simulink model "sf_tictacflow"  (R2017b)
settings: Solver=VariableStepDiscrete  StartTime=0.0  StopTime=inf  RelTol=1e-3  EnableMultiTasking=on
settings Model: FPTRunName=Active  ExtModeTrigMode=oneshot  ExtModeArmWhenConnect=off  ExtModeAutoUpdateStatusClock=off  Creator=The MathWorks, Inc.  LastModifiedBy=The MathWorks, Inc.
settings DataIOCC: SaveFormat=Array  SaveOutput=off  SaveTime=off  SignalLoggingName=sigsOut
settings OptimizationCC: BlockReduction=off  BooleanDataType=off  ExpressionDepthLimit=2147483647  InitFltsAndDblsToZero=on  EfficientMapNaN2IntZero=off  LifeSpan=inf  BufferReusableBoundary=off
settings DebuggingCC: SaveWithParameterizedLinksMsg=none  UnderspecifiedInitializationDetection=Classic  MergeDetectMultiDrivingBlocksExec=none  SignalResolutionControl=TryResolveAllWithWarning  MultiTaskDSMMsg=warning  MultiTaskCondExecSysMsg=none  FcnCallInpInsideContextMsg=warning  BusObjectLabelMismatch=none  AllowSymbolicDim=off  StateNameClashWarn=warning  SFUnexpectedBacktrackingDiag=warning  SFInvalidInputDataAccessInChartInitDiag=none  SFNoUnconditionalDefaultTransitionDiag=warning  SFUndirectedBroadcastEventsDiag=none  SFExecutionAtInitializationDiag=none  SFMachineParentedDataDiag=none
settings HardwareCC: ProdBitPerPointer=32  ProdBitPerSizeT=32  ProdBitPerPtrDiffT=32  ProdLargestAtomicFloat=None  ProdIntDivRoundTo=Undefined  ProdEndianess=Unspecified  ProdWordSize=32  ProdHWDeviceType=32-bit Generic  TargetUnknown=on
settings ModelReferenceCC: PropagateSignalLabelsOutOfModel=off
settings SFSimCC: SFSimEcho=off  SimParseCustomCode=off
settings CodeAppCC: StateflowObjectComments=on
settings GRTTargetCC: TargetFcnLib=ansi_tfl_tmw.mat  TargetLangStandard=C89/C90 (ANSI)  GeneratePreprocessorConditionals=Disable all  CombineOutputUpdateFcns=off  GRTInterface=on
settings ConfigComp: CovMetricSettings=dcmtr  CovHtmlReporting=on  CovSaveCumulativeToWorkspaceVar=on  CovSaveSingleToWorkspaceVar=on  CovExternalEMLEnable=off  CovSFcnEnable=off

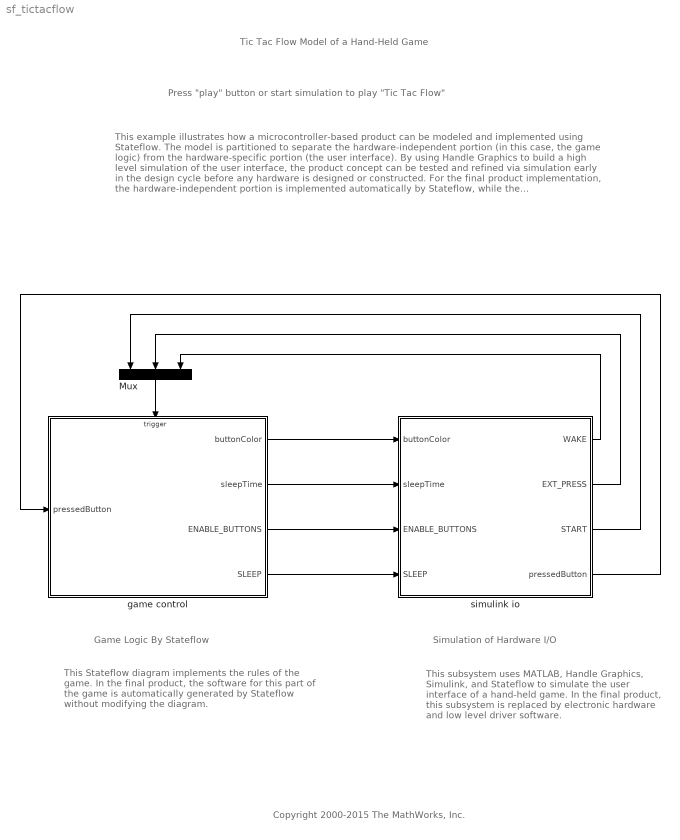
== system sf_tictacflow ==
  note: Press "play" button or start simulation to play "Tic Tac Flow"
  note: This Stateflow diagram implements
      | the rules of the game.
      |
      | In the final product, the software for this
      | part of the game is automatically generated
      |  by Stateflow without modifying the diagram.
  note: Game Logic By Stateflow
  note: This subsystem uses MATLAB, Handle
      | Graphics, Simulink, and Stateflow
      |  to simulate the user interface of a
      | hand-held game.
      |
      | In the final product, this subsystem is
      | replaced by electronic hardware and
      | low level driver software.
  note: This example illustrates how a microcontroller-based product can be modeled and implemented using Stateflow.
      |
      | The model is partitioned to separate the hardware-independent portion (in
      | this case, the game logic) from the hardware-specific portion (the user interface).
      | By using Handle Graphics to build a high level simulation of the user interface, the product concept can
      |  be tested and refined via simulation early in the design cycle before any hardware is designed or constructed.
      | For the final product implementation, the hardware-independent portion is implemented automatically
      |  by Stateflow, while the hardware-specific portion is replaced by actual hardware and low-level driver software.
  note: Tic Tac Flow
      | Model of a Hand-Held Game
  note: Simulation of Hardware I/O
  note: Copyright 2000-2015 The MathWorks, Inc.
  Mux : Mux  Inputs=3
  game control : Stateflow chart  TreatAsAtomicUnit=on
  simulink io : Subsystem  StopFcn=fig = findobj(0, 'Name', 'Tic Tac Flow'); if ishandle(fig); delete(fig); end;
  wires:
  Mux/1 -> game control/Trigger
  game control/2(sleepTime) -> simulink io/2(sleepTime)
  game control/3(ENABLE_BUTTONS) -> simulink io/3(ENABLE_BUTTONS)
  game control/4(SLEEP) -> simulink io/4(SLEEP)
  game control/1(buttonColor) -> simulink io/1(buttonColor)
  simulink io/1(WAKE) -> Mux/3
  simulink io/2(EXT_PRESS) -> Mux/2
  simulink io/3(START) -> Mux/1
  simulink io/4(pressedButton) -> game control/1(pressedButton)

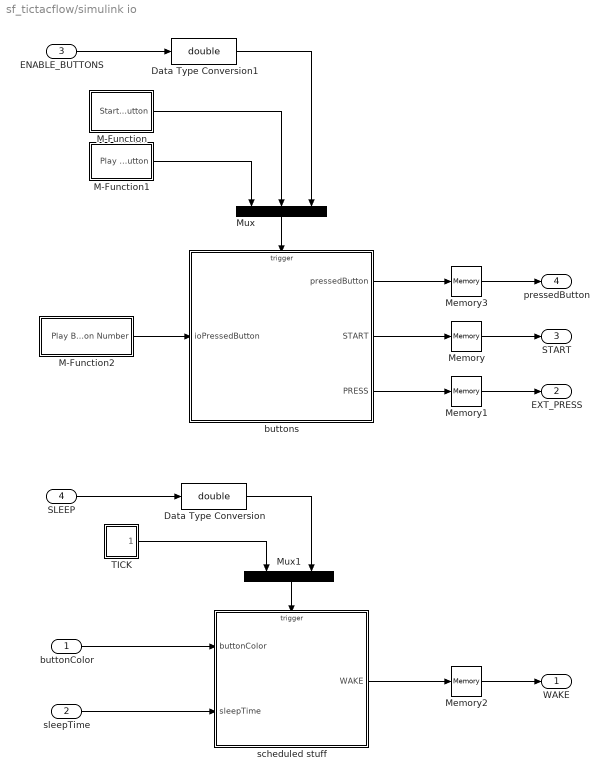
== system sf_tictacflow/simulink io ==
  buttonColor : Inport
  sleepTime : Inport  Port=2
  ENABLE_BUTTONS : Inport  Port=3
  SLEEP : Inport  Port=4
  Data Type Conversion : DataTypeConversion  OutDataTypeStr=double
  Data Type Conversion1 : DataTypeConversion  OutDataTypeStr=double
  M-Function : Subsystem
  M-Function1 : Subsystem
  M-Function2 : Subsystem
  Memory{,1..3} (4 alike) : Memory
  Mux : Mux  Inputs=3
  Mux1 : Mux  Inputs=2
  TICK : Subsystem  mask(Pulse Generator){period=1/60, duty=50, amplitude=1, start=0}
      mask prompts: period "Period (secs):"; duty "Duty cycle (% of period):"; start "Start time:"
      mask help: Pulse Generator
      mask Help: Pulse generator which ensures pulse transitions are hit. Provides a vector of pulses when the height is entered as a vector.  Unmask to see how it works.
      mask Display: plot(0,0,100,100,[95,90,90,75,75,60,60,45,45,30,30,15,15,5],[25,25,75,75,25,25,75,75,25,25,75,75,25,25]);
  buttons : Stateflow chart  TreatAsAtomicUnit=on
  scheduled stuff : Stateflow chart  TreatAsAtomicUnit=on
  WAKE : Outport
  EXT_PRESS : Outport  Port=2
  START : Outport  Port=3
  pressedButton : Outport  Port=4
  wires:
  Mux/1 -> buttons/Trigger
  Mux1/1 -> scheduled stuff/Trigger
  scheduled stuff/1(WAKE) -> Memory2/1
  Memory2/1 -> WAKE/1
  sleepTime/1 -> scheduled stuff/2(sleepTime)
  buttonColor/1 -> scheduled stuff/1(buttonColor)
  TICK/1(Out1) -> Mux1/1
  SLEEP/1 -> Data Type Conversion/1
  M-Function2/1(Play Button Number) -> buttons/1(ioPressedButton)
  M-Function1/1(Play Button) -> Mux/1
  M-Function/1(Start Button) -> Mux/2
  ENABLE_BUTTONS/1 -> Data Type Conversion1/1
  buttons/1(pressedButton) -> Memory3/1
  buttons/2(START) -> Memory/1
  Memory/1 -> START/1
  buttons/3(PRESS) -> Memory1/1
  Memory1/1 -> EXT_PRESS/1
  Memory3/1 -> pressedButton/1
  Data Type Conversion/1 -> Mux1/2
  Data Type Conversion1/1 -> Mux/3

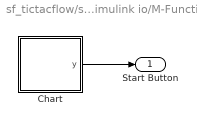
== system sf_tictacflow/simulink io/M-Function ==
  Chart : Stateflow chart  TreatAsAtomicUnit=on
  Start Button : Outport
  wires:
  Chart/1(y) -> Start Button/1

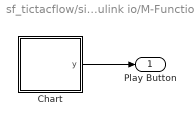
== system sf_tictacflow/simulink io/M-Function1 ==
  Chart : Stateflow chart  TreatAsAtomicUnit=on
  Play Button : Outport
  wires:
  Chart/1(y) -> Play Button/1

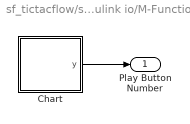
== system sf_tictacflow/simulink io/M-Function2 ==
  Chart : Stateflow chart  TreatAsAtomicUnit=on
  Play Button Number : Outport
  wires:
  Chart/1(y) -> Play Button Number/1

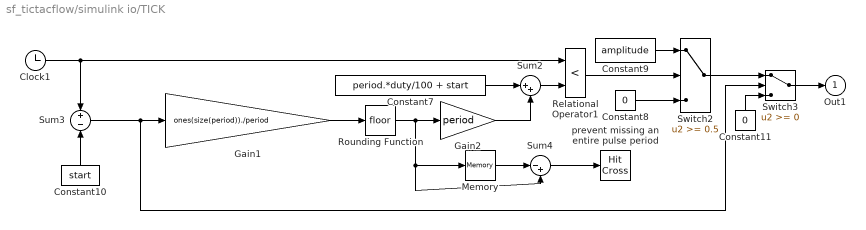
== system sf_tictacflow/simulink io/TICK ==
  Clock1 : Clock
  Constant10 : Constant  Value=start
  Constant11 : Constant  Value=0
  Constant7 : Constant  Value=period.*duty/100 + start
  Constant8 : Constant  Value=0
  Constant9 : Constant  Value=amplitude
  Gain1 : Gain  Gain=ones(size(period))./period  SaturateOnIntegerOverflow=on  OutDataTypeStr=Inherit: Same as input  ParamDataTypeStr=Inherit: Same as input
  Gain2 : Gain  Gain=period  SaturateOnIntegerOverflow=on  OutDataTypeStr=Inherit: Same as input  ParamDataTypeStr=Inherit: Same as input
  Memory : Memory
  Relational Operator1 : RelationalOperator  Operator=<  RndMeth=Nearest  InputSameDT=on
  Rounding Function : Rounding
  Sum2 : Sum  Inputs=|++  SaturateOnIntegerOverflow=on  InputSameDT=on  OutDataTypeStr=Inherit: Same as first input
  Sum3 : Sum  Inputs=+-  SaturateOnIntegerOverflow=on  InputSameDT=on  OutDataTypeStr=Inherit: Same as first input
  Sum4 : Sum  Inputs=|-+  SaturateOnIntegerOverflow=on  InputSameDT=on  OutDataTypeStr=Inherit: Same as first input
  Switch2 : Switch  Threshold=0.5  SaturateOnIntegerOverflow=on  InputSameDT=on
  Switch3 : Switch  SaturateOnIntegerOverflow=on  InputSameDT=on
  prevent missing an entire pulse period : HitCross  HitCrossingOffset=1  ShowOutputPort=off
  Out1 : Outport
  wires:
  Memory/1 -> Sum4/1
  Sum4/1 -> prevent missing an entire pulse period/1
  Switch2/1 -> Switch3/1
  Constant11/1 -> Switch3/3
  Constant9/1 -> Switch2/1
  Constant8/1 -> Switch2/3
  Relational Operator1/1 -> Switch2/2
  Switch3/1 -> Out1/1
  Rounding Function/1 -> Gain2/1, Memory/1, Sum4/2
  Gain2/1 -> Sum2/2
  Constant7/1 -> Sum2/1
  Gain1/1 -> Rounding Function/1
  Sum2/1 -> Relational Operator1/2
  Clock1/1 -> Sum3/1, Relational Operator1/1
  Sum3/1 -> Switch3/2, Gain1/1
  Constant10/1 -> Sum3/2

== stateflow chart sf_tictacflow/game control ==
  settings: executeAtInitialization=1
  state button_7 [parallel]
    settings: executionOrder=1
    state disabled
    state enabled
      buttonColor[thisButton] = DARK;
    state active
      state red
        buttonColor[thisButton] = RED;
        TURN;
      state green
        buttonColor[thisButton] = GREEN;
        TURN;
      (junction 226) -> button_7.active.red [order 2]
      (junction 226) -> button_7.active.green [order 1] : [in(turn.green)]
    button_7 -> (junction 230) : START
    (default) -> (junction 230)
    (junction 230) -> button_7.enabled
    button_7.enabled -> button_7.disabled [order 1] : GAME_OVER
    button_7.active.red -> button_7.disabled : GAME_OVER [in(turn.green)]
        | {buttonColor[thisButton] = DIM_RED; }
    button_7.active.green -> button_7.disabled : GAME_OVER [in(turn.red)]
        | {buttonColor[thisButton] = DIM_GREEN; }
    button_7.active -> button_7.enabled : at(7,TURN)
    button_7.enabled -> (junction 226) [order 2] : PRESS
  state button_0 [parallel]
    settings: executionOrder=2
    state disabled
    state enabled
      buttonColor[thisButton] = DARK;
    state active
      state red
        buttonColor[thisButton] = RED;
        TURN;
      state green
        buttonColor[thisButton] = GREEN;
        TURN;
      (junction 249) -> button_0.active.red [order 2]
      (junction 249) -> button_0.active.green [order 1] : [in(turn.green)]
    button_0 -> (junction 248) : START
    (default) -> (junction 248)
    (junction 248) -> button_0.enabled
    button_0.enabled -> button_0.disabled [order 1] : GAME_OVER
    button_0.active.red -> button_0.disabled : GAME_OVER [in(turn.green)]
        | {buttonColor[thisButton] = DIM_RED; }
    button_0.active.green -> button_0.disabled : GAME_OVER [in(turn.red)]
        | {buttonColor[thisButton] = DIM_GREEN; }
    button_0.active -> button_0.enabled : at(7,TURN)
    button_0.enabled -> (junction 249) [order 2] : PRESS
  state button_5 [parallel]
    settings: executionOrder=3
    state disabled
    state enabled
      buttonColor[thisButton] = DARK;
    state active
      state red
        buttonColor[thisButton] = RED;
        TURN;
      state green
        buttonColor[thisButton] = GREEN;
        TURN;
      (junction 251) -> button_5.active.red [order 2]
      (junction 251) -> button_5.active.green [order 1] : [in(turn.green)]
    button_5 -> (junction 250) : START
    (default) -> (junction 250)
    (junction 250) -> button_5.enabled
    button_5.enabled -> button_5.disabled [order 1] : GAME_OVER
    button_5.active.red -> button_5.disabled : GAME_OVER [in(turn.green)]
        | {buttonColor[thisButton] = DIM_RED; }
    button_5.active.green -> button_5.disabled : GAME_OVER [in(turn.red)]
        | {buttonColor[thisButton] = DIM_GREEN; }
    button_5.active -> button_5.enabled : at(7,TURN)
    button_5.enabled -> (junction 251) [order 2] : PRESS
  state button_2 [parallel]
    settings: executionOrder=4
    state disabled
    state enabled
      buttonColor[thisButton] = DARK;
    state active
      state red
        buttonColor[thisButton] = RED;
        TURN;
      state green
        buttonColor[thisButton] = GREEN;
        TURN;
      (junction 257) -> button_2.active.red [order 2]
      (junction 257) -> button_2.active.green [order 1] : [in(turn.green)]
    button_2 -> (junction 256) : START
    (default) -> (junction 256)
    (junction 256) -> button_2.enabled
    button_2.enabled -> button_2.disabled [order 1] : GAME_OVER
    button_2.active.red -> button_2.disabled : GAME_OVER [in(turn.green)]
        | {buttonColor[thisButton] = DIM_RED; }
    button_2.active.green -> button_2.disabled : GAME_OVER [in(turn.red)]
        | {buttonColor[thisButton] = DIM_GREEN; }
    button_2.active -> button_2.enabled : at(7,TURN)
    button_2.enabled -> (junction 257) [order 2] : PRESS
  state button_4 [parallel]
    settings: executionOrder=5
    state disabled
    state enabled
      buttonColor[thisButton] = DARK;
    state active
      state red
        buttonColor[thisButton] = RED;
        TURN;
      state green
        buttonColor[thisButton] = GREEN;
        TURN;
      (junction 255) -> button_4.active.red [order 2]
      (junction 255) -> button_4.active.green [order 1] : [in(turn.green)]
    button_4 -> (junction 254) : START
    (default) -> (junction 254)
    (junction 254) -> button_4.enabled
    button_4.enabled -> button_4.disabled [order 1] : GAME_OVER
    button_4.active.red -> button_4.disabled : GAME_OVER [in(turn.green)]
        | {buttonColor[thisButton] = DIM_RED; }
    button_4.active.green -> button_4.disabled : GAME_OVER [in(turn.red)]
        | {buttonColor[thisButton] = DIM_GREEN; }
    button_4.active -> button_4.enabled : at(7,TURN)
    button_4.enabled -> (junction 255) [order 2] : PRESS
  state button_6 [parallel]
    settings: executionOrder=6
    state disabled
    state enabled
      buttonColor[thisButton] = DARK;
    state active
      state red
        buttonColor[thisButton] = RED;
        TURN;
      state green
        buttonColor[thisButton] = GREEN;
        TURN;
      (junction 253) -> button_6.active.red [order 2]
      (junction 253) -> button_6.active.green [order 1] : [in(turn.green)]
    button_6 -> (junction 252) : START
    (default) -> (junction 252)
    (junction 252) -> button_6.enabled
    button_6.enabled -> button_6.disabled [order 1] : GAME_OVER
    button_6.active.red -> button_6.disabled : GAME_OVER [in(turn.green)]
        | {buttonColor[thisButton] = DIM_RED; }
    button_6.active.green -> button_6.disabled : GAME_OVER [in(turn.red)]
        | {buttonColor[thisButton] = DIM_GREEN; }
    button_6.active -> button_6.enabled : at(7,TURN)
    button_6.enabled -> (junction 253) [order 2] : PRESS
  state button_3 [parallel]
    settings: executionOrder=7
    state disabled
    state enabled
      buttonColor[thisButton] = DARK;
    state active
      state red
        buttonColor[thisButton] = RED;
        TURN;
      state green
        buttonColor[thisButton] = GREEN;
        TURN;
      (junction 263) -> button_3.active.red [order 2]
      (junction 263) -> button_3.active.green [order 1] : [in(turn.green)]
    button_3 -> (junction 262) : START
    (default) -> (junction 262)
    (junction 262) -> button_3.enabled
    button_3.enabled -> button_3.disabled [order 1] : GAME_OVER
    button_3.active.red -> button_3.disabled : GAME_OVER [in(turn.green)]
        | {buttonColor[thisButton] = DIM_RED; }
    button_3.active.green -> button_3.disabled : GAME_OVER [in(turn.red)]
        | {buttonColor[thisButton] = DIM_GREEN; }
    button_3.active -> button_3.enabled : at(7,TURN)
    button_3.enabled -> (junction 263) [order 2] : PRESS
  state button_8 [parallel]
    settings: executionOrder=8
    state disabled
    state enabled
      buttonColor[thisButton] = DARK;
    state active
      state red
        buttonColor[thisButton] = RED;
        TURN;
      state green
        buttonColor[thisButton] = GREEN;
        TURN;
      (junction 261) -> button_8.active.red [order 2]
      (junction 261) -> button_8.active.green [order 1] : [in(turn.green)]
    button_8 -> (junction 260) : START
    (default) -> (junction 260)
    (junction 260) -> button_8.enabled
    button_8.enabled -> button_8.disabled [order 1] : GAME_OVER
    button_8.active.red -> button_8.disabled : GAME_OVER [in(turn.green)]
        | {buttonColor[thisButton] = DIM_RED; }
    button_8.active.green -> button_8.disabled : GAME_OVER [in(turn.red)]
        | {buttonColor[thisButton] = DIM_GREEN; }
    button_8.active -> button_8.enabled : at(7,TURN)
    button_8.enabled -> (junction 261) [order 2] : PRESS
  state button_1 [parallel]
    settings: executionOrder=9
    state disabled
    state enabled
      buttonColor[thisButton] = DARK;
    state active
      state red
        buttonColor[thisButton] = RED;
        TURN;
      state green
        buttonColor[thisButton] = GREEN;
        TURN;
      (junction 259) -> button_1.active.red [order 2]
      (junction 259) -> button_1.active.green [order 1] : [in(turn.green)]
    button_1 -> (junction 258) : START
    (default) -> (junction 258)
    (junction 258) -> button_1.enabled
    button_1.enabled -> button_1.disabled [order 1] : GAME_OVER
    button_1.active.red -> button_1.disabled : GAME_OVER [in(turn.green)]
        | {buttonColor[thisButton] = DIM_RED; }
    button_1.active.green -> button_1.disabled : GAME_OVER [in(turn.red)]
        | {buttonColor[thisButton] = DIM_GREEN; }
    button_1.active -> button_1.enabled : at(7,TURN)
    button_1.enabled -> (junction 259) [order 2] : PRESS
  state turn [parallel]
    settings: executionOrder=10
    state red
      buttonColor[9] = RED;
      ENABLE_BUTTONS;
    state move = choose_move() [function]
      (default) -> (junction 223) : /* try to win on this move */
          | { move = 12 - gameState[1] - gameState[3]; }
      (junction 223) -> (junction 218) [order 1] : [ make_move_if_available(move) ]
      (junction 223) -> (junction 217) [order 2] : /* else try to block opponent from winning next move */
          | { move = 12 - gameState[0] - gameState[2]; }
      (junction 217) -> (junction 235) [order 1] : [ make_move_if_available(move) ]
      (junction 217) -> (junction 227) [order 2] : /* else make a random  move */
          | { move = seed; }
      (junction 238) -> (junction 227)
      (junction 227) -> (junction 219) : {
          |   /* simple linear congruential
          |      pseudo-random sequence:
          |      x = (5x + 3) mod 16 */
          |   move += move << 2;
          |   move += 3;
          |   move &= 0xf;
          | }
      (junction 239) -> (junction 238)
      (junction 219) -> (junction 239) [order 1] : [!make_move_if_available(move)]
      (junction 219) -> (junction 213) [order 2] : { seed = move; }
    state shift_game_state(magicNumber) [function]
      (default) -> (junction 231) : {
          |   gameState[5] = gameState[4];
          |   gameState[4] = gameState[3];
          |   gameState[3] = gameState[2];
          |   gameState[2] = gameState[1];
          |   gameState[1] = gameState[0];
          |   gameState[0] = magicNumber;
          | }
    state game_over
    state yes = make_move_if_available(move) [function]
      (default) -> (junction 214)
      (junction 214) -> (junction 224) [order 1] : [ move == 0 && in(button_0.enabled)] { shift_game_state(move); send(PRESS,button_0);}
      (junction 214) -> (junction 212) [order 2]
      (junction 224) -> (junction 216)
      (junction 212) -> (junction 216) [order 1] : [ move == 1 && in(button_1.enabled)] { shift_game_state(move); send(PRESS,button_1);}
      (junction 212) -> (junction 234) [order 2]
      (junction 216) -> (junction 233)
      (junction 234) -> (junction 233) [order 1] : [ move == 2 && in(button_2.enabled)] { shift_game_state(move); send(PRESS,button_2);}
      (junction 234) -> (junction 220) [order 2]
      (junction 233) -> (junction 221)
      (junction 220) -> (junction 221) [order 1] : [ move == 3 && in(button_3.enabled)] { shift_game_state(move); send(PRESS,button_3);}
      (junction 220) -> (junction 247) [order 2]
      (junction 221) -> (junction 246)
      (junction 247) -> (junction 246) [order 1] : [ move == 4 && in(button_4.enabled)] { shift_game_state(move); send(PRESS,button_4);}
      (junction 247) -> (junction 245) [order 2]
      (junction 246) -> (junction 244)
      (junction 245) -> (junction 244) [order 1] : [ move == 5 && in(button_5.enabled)] { shift_game_state(move); send(PRESS,button_5);}
      (junction 245) -> (junction 243) [order 2]
      (junction 244) -> (junction 242)
      (junction 243) -> (junction 242) [order 1] : [ move == 6 && in(button_6.enabled)] { shift_game_state(move); send(PRESS,button_6);}
      (junction 243) -> (junction 241) [order 2]
      (junction 242) -> (junction 240)
      (junction 241) -> (junction 240) [order 1] : [ move == 7 && in(button_7.enabled)] { shift_game_state(move); send(PRESS,button_7);}
      (junction 241) -> (junction 232) [order 2]
      (junction 240) -> (junction 222)
      (junction 232) -> (junction 222) [order 1] : [ move == 8 && in(button_8.enabled)] { shift_game_state(move); send(PRESS,button_8);}
      (junction 232) -> (junction 229) [order 2] : { yes = 0; }
      (junction 222) -> (junction 236) : { yes = 1; }
    state yes = is_a_winner() [function]
      (default) -> (junction 225) : { yes =((gameState[0] + gameState[2] + gameState[4]) == 12); }
    state green
      buttonColor[9] = GREEN;
      state sleeping
        sleepTime = 255;
        SLEEP;
      state two_player
        ENABLE_BUTTONS;
      state awakened
        choose_move();
      (default) -> (junction 264)
      (junction 264) -> two_player [order 1] : [TWO_PLAYER]
      (junction 264) -> sleeping [order 2]
      sleeping -> awakened : WAKE
    turn -> (junction 265) [order 1] : EXT_PRESS
    turn -> (junction 215) [order 2] : START
    (default) -> (junction 215)
    (junction 265) -> (junction 266) [order 1] : [ make_move_if_available( pressedButton ) ]
    (junction 265) -> (junction 267) [order 2] : { ENABLE_BUTTONS; }
    (junction 215) -> turn.red : { gameState = 13; }
    (junction 237) -> turn.red [order 2]
    turn.red -> (junction 228) : TURN
    (junction 228) -> game_over [order 1] : [is_a_winner()] {GAME_OVER; }
    (junction 237) -> game_over [order 1] : [is_a_winner()] {GAME_OVER;}
    turn.green -> (junction 237) : TURN
    (junction 228) -> turn.green [order 2]
  data: thisButton constant uint8 =7; thisButton constant uint8; thisButton constant uint8 =5; thisButton constant uint8 =2; thisButton constant uint8 =4; thisButton constant uint8 =6; thisButton constant uint8 =3; thisButton constant uint8 =8; thisButton constant uint8 =1; move function_output int8; magicNumber function_input uint8; move function_input int8; yes function_output boolean; yes function_output boolean; gameState local int8 size=9; seed local uint8 =13; RED constant uint8 =15; DIM_RED constant uint8 =8; GREEN constant uint8 =240; DIM_GREEN constant uint8 =128; DARK constant uint8; TWO_PLAYER constant boolean; buttonColor output uint8 size=10; sleepTime output uint8; pressedButton input uint8
  events: TURN local EITHER_EDGE_EVENT; GAME_OVER local EITHER_EDGE_EVENT; ENABLE_BUTTONS output EITHER_EDGE_EVENT; START input EITHER_EDGE_EVENT; EXT_PRESS input EITHER_EDGE_EVENT; PRESS local EITHER_EDGE_EVENT; SLEEP output EITHER_EDGE_EVENT; WAKE input EITHER_EDGE_EVENT

== stateflow chart sf_tictacflow/simulink io/buttons ==
  settings: sampleTime=1  executeAtInitialization=1
  state io [parallel]
    en:
    figH = ml.sf_tictacflowgui('fig');
    ml.set(figH,'Pointer','arrow');
    /* note mapping between magic numbers and button location:
    buttonH[magic] = ml.play_button_magic(figH,location,magic);  */
    buttonH0 = ml.sf_tictacflowgui('play_button',figH,1,0);
    buttonH1 = ml.sf_tictacflowgui('play_button',figH,8,1);
    buttonH2 = ml.sf_tictacflowgui('play_button',figH,3,2);
    buttonH3 = ml.sf_tictacflowgui('play_button',figH,6,3);
    buttonH4 = ml.sf_tictacflowgui('play_button',figH,4,4);
    buttonH5 = ml.sf_tictacflowgui('play_button',figH,2,5);
    buttonH6 = ml.sf_tictacflowgui('play_button',figH,5,6);
    buttonH7 = ml.sf_tictacflowgui('play_button',figH,0,7);
    buttonH8 = ml.sf_tictacflowgui('play_button',figH,7,8);
    startButtonH = ml.sf_tictacflowgui('start_button',figH);
    turnSignalH = ml.sf_tictacflowgui('turn_signal',figH);
    settings: executionOrder=1
    io -> (junction 13)
    (junction 13) -> (junction 11) [order 1] : IO_START
        | {
        |    pressedButton = 0;
        |    START;
        | }
    (junction 13) -> (junction 14) [order 2]
    (junction 14) -> (junction 10) [order 1] : ENABLE_BUTTONS
        | {
        |   ml.set(buttonH0,'Enable','On');
        |   ml.set(buttonH1,'Enable','On');
        |   ml.set(buttonH2,'Enable','On');
        |   ml.set(buttonH3,'Enable','On');
        |   ml.set(buttonH4,'Enable','On');
        |   ml.set(buttonH5,'Enable','On');
        |   ml.set(buttonH6,'Enable','On');
        |   ml.set(buttonH7,'Enable','On');
        |   ml.set(buttonH8,'Enable','On');
        | }
    (junction 14) -> (junction 15) [order 2]
    (junction 15) -> (junction 12) [order 1] : IO_PRESS
        | {
        |   ml.set(buttonH0,'Enable','Off');
        |   ml.set(buttonH1,'Enable','Off');
        |   ml.set(buttonH2,'Enable','Off');
        |   ml.set(buttonH3,'Enable','Off');
        |   ml.set(buttonH4,'Enable','Off');
        |   ml.set(buttonH5,'Enable','Off');
        |   ml.set(buttonH6,'Enable','Off');
        |   ml.set(buttonH7,'Enable','Off');
        |   ml.set(buttonH8,'Enable','Off');
        |   pressedButton = ioPressedButton;
        |   PRESS;
        | }
    (junction 15) -> (junction 9) [order 2]
  data: startButtonH local ml; ioPressedButton input double; pressedButton output uint8
  events: IO_PRESS input EITHER_EDGE_EVENT; IO_START input EITHER_EDGE_EVENT; ENABLE_BUTTONS input EITHER_EDGE_EVENT; START output EITHER_EDGE_EVENT; PRESS output EITHER_EDGE_EVENT

== stateflow chart sf_tictacflow/simulink io/scheduled stuff ==
  settings: sampleTime=1  executeAtInitialization=1
  state stop [parallel]
    settings: executionOrder=1
    stop -> (junction 17)
    (default) -> (junction 17)
    (junction 17) -> (junction 16) : [ !ml.ishandle(figH) ]
        | { ml.set_param('sf_tictacflow','simulationcommand','stop'); }
  state update_LEDs [parallel]
    settings: executionOrder=2
    update_LEDs -> (junction 18)
    (default) -> (junction 18)
    (junction 18) -> (junction 15) : TICK
        | [ml.ishandle(figH)]
        | {
        |   ml.sf_tictacflowgui('set_button_color',buttonH0,buttonColor[0]);
        |   ml.sf_tictacflowgui('set_button_color',buttonH1,buttonColor[1]);
        |   ml.sf_tictacflowgui('set_button_color',buttonH2,buttonColor[2]);
        |   ml.sf_tictacflowgui('set_button_color',buttonH3,buttonColor[3]);
        |   ml.sf_tictacflowgui('set_button_color',buttonH4,buttonColor[4]);
        |   ml.sf_tictacflowgui('set_button_color',buttonH5,buttonColor[5]);
        |   ml.sf_tictacflowgui('set_button_color',buttonH6,buttonColor[6]);
        |   ml.sf_tictacflowgui('set_button_color',buttonH7,buttonColor[7]);
        |   ml.sf_tictacflowgui('set_button_color',buttonH8,buttonColor[8]);
        |   ml.sf_tictacflowgui('set_button_color',turnSignalH,buttonColor[9]);
        | }
  state sleep [parallel]
    settings: executionOrder=3
    state awake
    state asleep
      entry:
      ml.set(figH,'Pointer','watch');
      exit:
      ml.set(figH,'Pointer','arrow');
    (default) -> awake
    awake -> asleep : SLEEP
    asleep -> awake : after(sleepTime,TICK)
        | { WAKE; }
  data: buttonColor input uint8 size=10; sleepTime input uint8
  events: TICK input EITHER_EDGE_EVENT; SLEEP input EITHER_EDGE_EVENT; WAKE output EITHER_EDGE_EVENT

== stateflow chart sf_tictacflow/simulink io/M-Function1/Chart ==
  (default) -> (junction 2) : {y = ml.sf_tictacflowgui(1);}
  data: y output double

== stateflow chart sf_tictacflow/simulink io/M-Function2/Chart ==
  (default) -> (junction 2) : {y = ml.sf_tictacflowgui(2);}
  data: y output double

== stateflow chart sf_tictacflow/simulink io/M-Function/Chart ==
  (default) -> (junction 2) : {y = ml.sf_tictacflowgui(0);}
  data: y output double
